simulink model "Vfinal"  (R2023a)
settings: Solver=VariableStepAuto  StartTime=0.0  StopTime=10.0  RelTol=1e-3
settings Model: Creator=meghn  LastModifiedBy=meghn

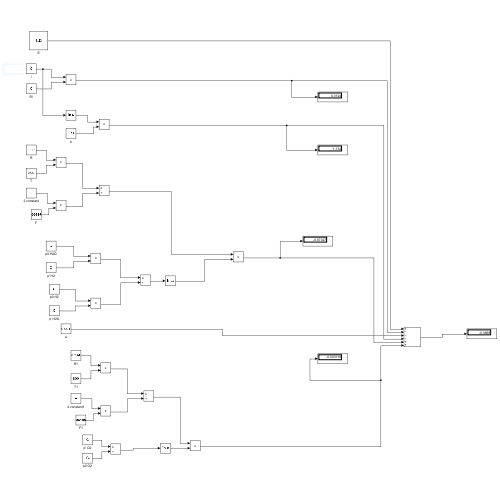
[thumbnail: Simulink's stored preview of the top-level diagram]
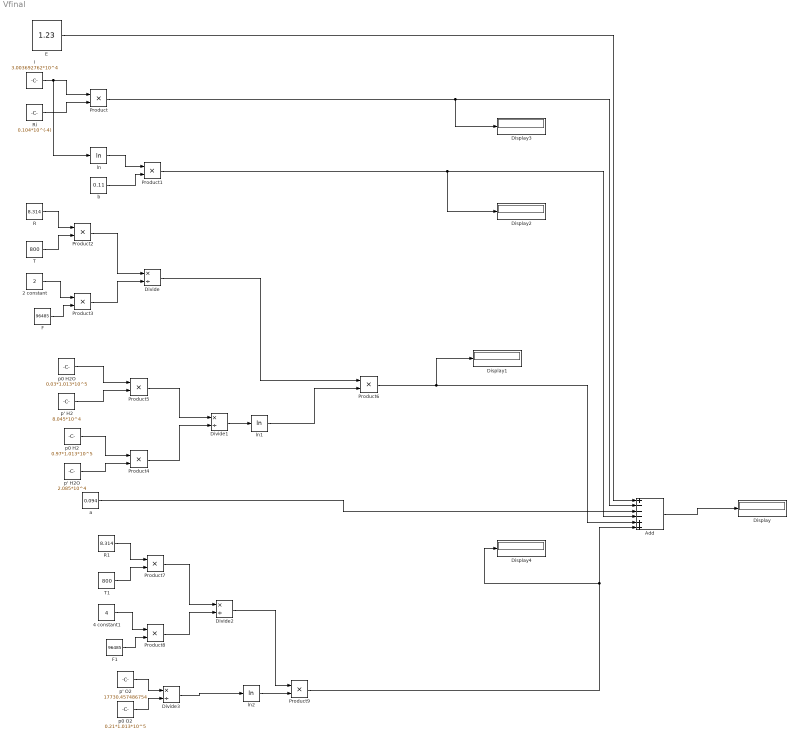
== system Vfinal ==
  2 constant : Constant  Value=2
  4 constant1 : Constant  Value=4
  Add : Sum  Inputs=+---++
  Display{,1..4} (5 alike) : Display
  Divide{,1..3} (4 alike) : Product  Inputs=*/
  E : Constant  Value=1.23
  F : Constant  Value=96485
  F1 : Constant  Value=96485
  Product{,1..9} (10 alike) : Product
  R : Constant  Value=8.314
  R1 : Constant  Value=8.314
  Ri : Constant  Value=0.104*10^(-4)
  T : Constant  Value=800
  T1 : Constant  Value=800
  a : Constant  Value=0.094
  b : Constant  Value=0.11
  i : Constant  Value=3.003692762*10^4
  ln : Math  Operator=log
  ln1 : Math  Operator=log
  ln2 : Math  Operator=log
  p' H2 : Constant  Value=8.045*10^4
  p' H2O : Constant  Value=2.085*10^4
  p' O2 : Constant  Value=17730.457486754
  p0 H2 : Constant  Value=0.97*1.013*10^5
  p0 H2O : Constant  Value=0.03*1.013*10^5
  p0 O2 : Constant  Value=0.21*1.013*10^5
  wires:
  i/1 -> ln/1, Product/1
  Ri/1 -> Product/2
  ln/1 -> Product1/1
  b/1 -> Product1/2
  R/1 -> Product2/1
  T/1 -> Product2/2
  2 constant/1 -> Product3/1
  F/1 -> Product3/2
  Product2/1 -> Divide/1
  Product3/1 -> Divide/2
  p' H2/1 -> Product5/2
  p' H2O/1 -> Product4/2
  Product5/1 -> Divide1/1
  p0 H2/1 -> Product4/1
  Product4/1 -> Divide1/2
  Divide1/1 -> ln1/1
  p0 H2O/1 -> Product5/1
  Divide/1 -> Product6/1
  ln1/1 -> Product6/2
  R1/1 -> Product7/1
  T1/1 -> Product7/2
  Product8/1 -> Divide2/2
  Product7/1 -> Divide2/1
  F1/1 -> Product8/2
  4 constant1/1 -> Product8/1
  p' O2/1 -> Divide3/1
  p0 O2/1 -> Divide3/2
  Divide3/1 -> ln2/1
  Divide2/1 -> Product9/1
  ln2/1 -> Product9/2
  E/1 -> Add/1
  Product/1 -> Display3/1, Add/2
  a/1 -> Add/3
  Product9/1 -> Display4/1, Add/6
  Product6/1 -> Display1/1, Add/5
  Product1/1 -> Display2/1, Add/4
  Add/1 -> Display/1
